simulink model "interpprueba"  (R2021b)
settings: Solver=VariableStepAuto  StartTime=0.0  StopTime=10.0  RelTol=1e-3
values from neighbouring files (symbols this model uses):
  fp = [t1;t2;t3]    [creacionestructurasborrador.m]    (also in flight_plan.m = [sid,wps,iap]; flight_plan_eval.m = [t1;tabla2;t3]; flight_plan_old.m = [sid,wps,iap]; flight_plan_struct.m = [t1;tabla2;t3])
settings Model: Creator=verti  LastModifiedBy=verti

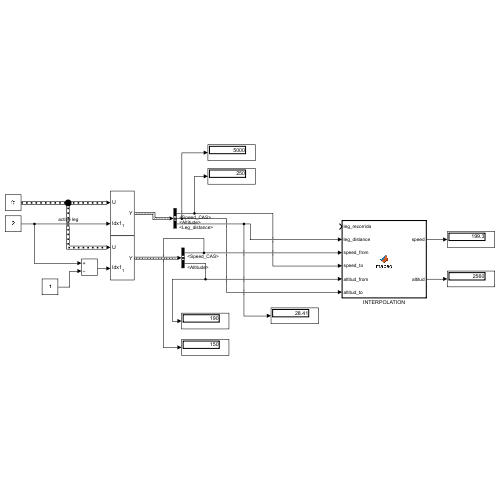
[thumbnail: Simulink's stored preview of the top-level diagram]
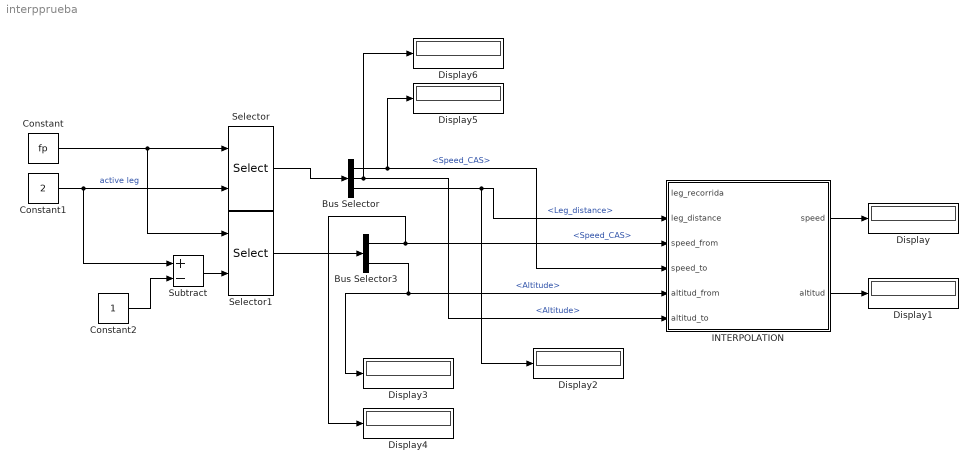
== system interpprueba ==
  Bus Selector : BusSelector  RequirementInfo={} %GIDa_748c13b4_26a4_4f06_b41f_6c0f351aa6e1  OutputSignals=Speed_CAS,Altitude,Leg_distance
  Bus Selector3 : BusSelector  RequirementInfo={} %GIDa_962e6f27_d2e9_4d95_8ffb_528ca1f04bd7  OutputSignals=Speed_CAS,Altitude
  Constant : Constant  Value=fp  OutDataTypeStr=Bus: BUS_FP
  Constant1 : Constant  Value=2
  Constant2 : Constant
  Display{,1..6} (7 alike) : Display
  INTERPOLATION : MATLAB Function  RequirementInfo={} %GIDa_00da5b89_cd18_4ad3_bdd9_46f4b2278232  TreatAsAtomicUnit=on
  Selector : Selector  RequirementInfo={} %GIDa_52603b66_c8a4_4acb_b10d_5686338dd3d7  InputPortWidth=12  IndexOptions=Index vector (port)  Indices=[1 3]  OutputSizes=1
  Selector1 : Selector  RequirementInfo={} %GIDa_aadcde5b_c971_450e_aee0_b769e6a2f6d5  InputPortWidth=12  IndexOptions=Index vector (port)  Indices=[1 3]  OutputSizes=1
  Subtract : Sum  Inputs=+-
  wires:
  Bus Selector3/2 -> INTERPOLATION/5(altitud_from), Display3/1  "<Altitude>"
  Constant1/1 -> Subtract/1, Selector/2  "active leg"
  Constant/1 -> Selector/1, Selector1/1
  Subtract/1 -> Selector1/2
  Selector1/1 -> Bus Selector3/1
  Bus Selector/2 -> Display6/1, INTERPOLATION/6(altitud_to)  "<Altitude>"
  Selector/1 -> Bus Selector/1
  Bus Selector/1 -> Display5/1, INTERPOLATION/4(speed_to)  "<Speed_CAS>"
  Bus Selector3/1 -> Display4/1, INTERPOLATION/3(speed_from)  "<Speed_CAS>"
  Constant2/1 -> Subtract/2
  INTERPOLATION/1(speed) -> Display/1
  INTERPOLATION/2(altitud) -> Display1/1
  Bus Selector/3 -> Display2/1, INTERPOLATION/2(leg_distance)  "<Leg_distance>"

== matlab function interpprueba/INTERPOLATION ==
  data: leg_recorrida input; leg_distance input; speed_from input; speed_to input; altitud_from input; speed output; altitud_to input; altitud output
function [speed,altitud] = mapeo(leg_recorrida,leg_distance,speed_from,speed_to,altitud_from,altitud_to)

speed = (leg_recorrida) .* (speed_to - speed_from) ./ (leg_distance) + speed_from;
altitud = (leg_recorrida) .* (altitud_to - altitud_from) ./ (leg_distance) + altitud_from;

end
